simulink model "MotionSystemControl_2020b_TestINS_6DOF"  (R2020b)
settings: Solver=VariableStepAuto  StartTime=0.0  StopTime=165  RelTol=1e-3
libraries: MotionSystems_Simulink x7
settings Model: EnablePacing=on  Creator=usr  LastModifiedBy=yiyin

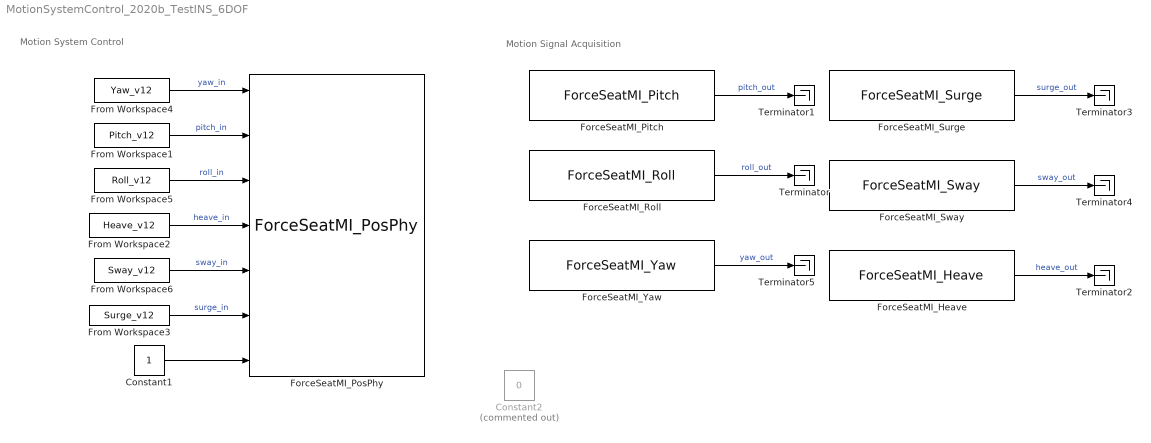
== system MotionSystemControl_2020b_TestINS_6DOF ==
  note: Motion System Control
  note: Motion Signal Acquisition
  Constant1 : Constant  OutDataTypeStr=int32
  Constant2 : Constant  Commented=on  Value=0
  ForceSeatMI_Heave : MotionSystems_Simulink/ForceSeatMI_Heave
      settings: SourceProductName=MotionsSystems ForceSeatMI
  ForceSeatMI_Pitch : MotionSystems_Simulink/ForceSeatMI_Pitch
      settings: SourceProductName=MotionsSystems ForceSeatMI
  ForceSeatMI_PosPhy : MotionSystems_Simulink/ForceSeatMI_PosPhy
  ForceSeatMI_Roll : MotionSystems_Simulink/ForceSeatMI_Roll
      settings: SourceProductName=MotionsSystems ForceSeatMI
  ForceSeatMI_Surge : MotionSystems_Simulink/ForceSeatMI_Surge
      settings: SourceProductName=MotionsSystems ForceSeatMI
  ForceSeatMI_Sway : MotionSystems_Simulink/ForceSeatMI_Sway
      settings: SourceProductName=MotionsSystems ForceSeatMI
  ForceSeatMI_Yaw : MotionSystems_Simulink/ForceSeatMI_Yaw
  From Workspace1 : FromWorkspace  VariableName=Pitch_v12  SampleTime=0.025
  From Workspace2 : FromWorkspace  VariableName=Heave_v12  SampleTime=0.025
  From Workspace3 : FromWorkspace  VariableName=Surge_v12  SampleTime=0.025
  From Workspace4 : FromWorkspace  VariableName=Yaw_v12  SampleTime=0.025
  From Workspace5 : FromWorkspace  VariableName=Roll_v12  SampleTime=0.025
  From Workspace6 : FromWorkspace  VariableName=Sway_v12  SampleTime=0.025
  Terminator{,1..5} (6 alike) : Terminator
  wires:
  Constant1/1 -> ForceSeatMI_PosPhy/7
  ForceSeatMI_Roll/1 -> Terminator/1  "roll_out"
  From Workspace1/1 -> ForceSeatMI_PosPhy/2  "pitch_in"
  ForceSeatMI_Pitch/1 -> Terminator1/1  "pitch_out"
  ForceSeatMI_Heave/1 -> Terminator2/1  "heave_out"
  ForceSeatMI_Surge/1 -> Terminator3/1  "surge_out"
  From Workspace2/1 -> ForceSeatMI_PosPhy/4  "heave_in"
  From Workspace3/1 -> ForceSeatMI_PosPhy/6  "surge_in"
  ForceSeatMI_Sway/1 -> Terminator4/1  "sway_out"
  ForceSeatMI_Yaw/1 -> Terminator5/1  "yaw_out"
  From Workspace4/1 -> ForceSeatMI_PosPhy/1  "yaw_in"
  From Workspace5/1 -> ForceSeatMI_PosPhy/3  "roll_in"
  From Workspace6/1 -> ForceSeatMI_PosPhy/5  "sway_in"
